simulink model "sampleModel124"  (R2021b)
settings: Solver=VariableStepAuto  StartTime=0.0  StopTime=10.0  RelTol=1e-3
undefined symbols (not defined in the file or in its folder): Newton, Raphson
libraries: simulink x7
settings Model: Creator=user  LastModifiedBy=user

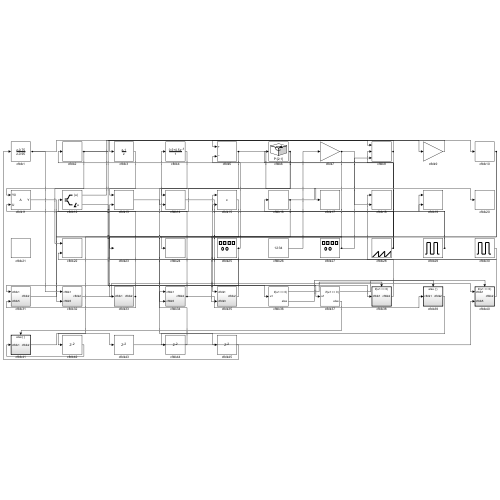
[thumbnail: Simulink's stored preview of the top-level diagram]
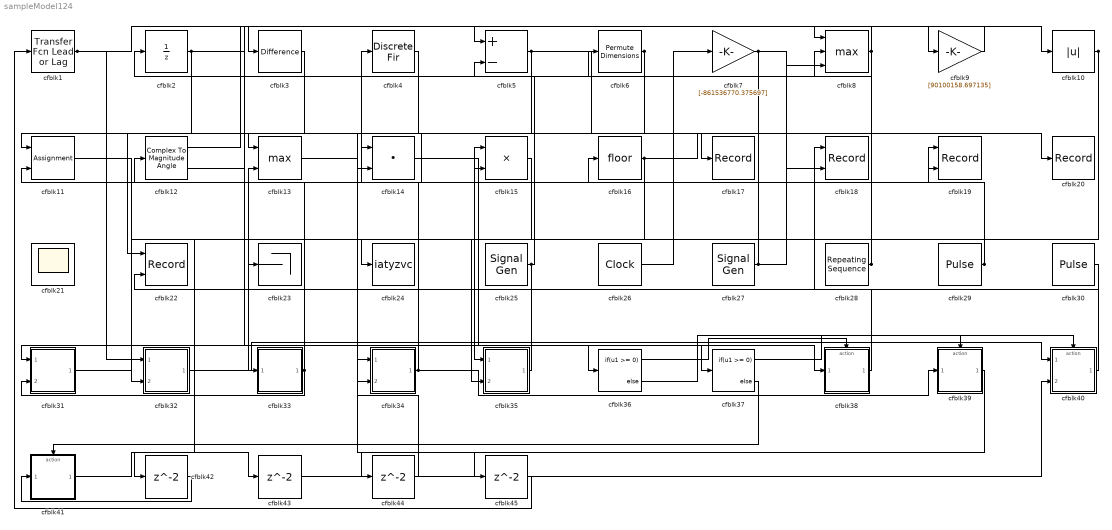
== system sampleModel124 ==
  cfblk1 : simulink/Discrete/Transfer Fcn Lead or Lag  PoleZ=0.95  ZeroZ=0.75  ICPrevOutput=0.0  ICPrevInput=0.0  DoSatur=off
      settings: SourceProductBaseCode=SL
  cfblk10 : Abs
  cfblk11 : Assignment  DiagnosticForDimensions=Warning  IndexOptions=Index vector (dialog)  Indices=1  OutputSizes=1
  cfblk12 : ComplexToMagnitudeAngle
  cfblk13 : MinMax  Function=max  Inputs=2
  cfblk14 : DotProduct  InputSameDT=on  OutDataTypeStr=Inherit: Inherit via internal rule
  cfblk15 : Product  Inputs=**
  cfblk16 : Rounding
  cfblk17 : Record  FileSettingsInternal="{\"entries\":[{\"content\":{\"excelSettings\":{\"content\":{},\"type\":\"Streamout.ExcelSettings\"}},\"type\":\"Streamout.FileSettingStorage\",\"uuid\":\"4b455be7-6192-4367-962d-3753fbca5225\"}],\"packageUris\":[\"http://schema.mathworks.com/mf0/streamout_blocks/R2020a\"],\"version\":\"1.0\"}"  SignalsInternal="{\"entries\":[{\"content\":{\"signals\":[{\"content\":{\"blockPath\":[\"sampleModel124/cfblk17\"],\"channel\":[],\"dimensions\":[1],\"domain\":\"sampleModel124/cfblk17\",\"lineColor\":\"#ff6929\",\"plots\":[1],\"port\":1,\"sid\":[\"\"],\"signalID\":4331,\"signalName\":\"cfblk5\"},\"type\":\"RecordBlkView.Signal\",\"uuid\":\"d4c4a8db-8163-4ec6-83a6-40b1eebb3f8b\"}]},\"type\":\"RecordBlkView.InputSignals\",\"uuid\":\"e1b93c3d-c5e7-46c7-8ecf-dc3223401c6b\"}],\"packageUris\":[\"http://schema.mathworks.com/mf0/streamout_blocks/R2020a\"],\"version\":\"1.0\"}"  VisualizationBindings="{\"sparklinesplugin\":{\"info\":[{\"bindingParametersList\":[],\"subplotID\":1}]}}"
  cfblk18 : Record  FileSettingsInternal="{\"entries\":[{\"content\":{\"excelSettings\":{\"content\":{},\"type\":\"Streamout.ExcelSettings\"}},\"type\":\"Streamout.FileSettingStorage\",\"uuid\":\"5ddf4468-bc94-43dd-8064-347963570ec6\"}],\"packageUris\":[\"http://schema.mathworks.com/mf0/streamout_blocks/R2020a\"],\"version\":\"1.0\"}"  Layout=[1 1]  SignalsInternal="{\"entries\":[{\"content\":{\"signals\":[{\"content\":{\"blockPath\":[\"sampleModel124/cfblk18\"],\"channel\":[],\"dimensions\":[1,1],\"domain\":\"sampleModel124/cfblk18\",\"lineColor\":\"#a2142f\",\"plots\":[1],\"port\":1,\"sid\":[\"\"],\"signalID\":4335,\"signalName\":\"cfblk38\"},\"type\":\"RecordBlkView.Signal\",\"uuid\":\"6f366cca-8914-4087-904e-589c9d18393c\"},{\"content\":{\"blockPath\":[\"sampleModel124/cfblk18\"],\"channel\":[],\"dimensions\":[1],\"domain\":\"sampleModel124/cfblk18\",\"lineColor\":\"#139fff\",\"plots\":[1],\"port\":2,\"sid\":[\"\"],\"signalID\":4339,\"signalName\":\"cfblk7\"},\"type\":\"RecordBlkView.Signal\",\"uuid\":\"3a6cb04f-8c68-44d5-8e53-ab1c3aa4fd33\"}]},\"type\":\"RecordBlkView.InputSignals\",\"uuid\":\"5846e25f-c3c2-42a3-b1e2-66c68f464335\"}],\"packageUris\":[\"http://schema.mathworks.com/mf0/streamout_blocks/R2020a\"],\"version\":\"1.0\"}"  VisualizationBindings="{\"xyplotplugin\":{\"info\":[{\"series\":[{\"bindingParametersList\":[{\"parameter\":\"X-Axis\",\"signalID\":4335,\"signalName\":\"cfblk38\"},{\"parameter\":\"Y-Axis\",\"signalID\":4339,\"signalName\":\"cfblk7\"}],\"seriesID\":22074}],\"subplotID\":1}]}}"  CompatibilityTag=XY
  cfblk19 : Record  FileSettingsInternal="{\"entries\":[{\"content\":{\"excelSettings\":{\"content\":{},\"type\":\"Streamout.ExcelSettings\"}},\"type\":\"Streamout.FileSettingStorage\",\"uuid\":\"7b857b01-50db-48e1-8f6f-10bc7bf9b4dc\"}],\"packageUris\":[\"http://schema.mathworks.com/mf0/streamout_blocks/R2020a\"],\"version\":\"1.0\"}"  Layout=[1 1]  SignalsInternal="{\"entries\":[{\"content\":{\"signals\":[{\"content\":{\"blockPath\":[\"sampleModel124/cfblk19\"],\"channel\":[],\"dimensions\":[1],\"domain\":\"sampleModel124/cfblk19\",\"lineColor\":\"#a2142f\",\"plots\":[1],\"port\":1,\"sid\":[\"\"],\"signalID\":4343,\"signalName\":\"cfblk31\"},\"type\":\"RecordBlkView.Signal\",\"uuid\":\"19b1038e-ab8c-450c-ab49-0e94919ec1bc\"},{\"content\":{\"blockPath\":[\"sampleModel124/cfblk19\"],\"channel\":[],\"dimensions\":[1],\"domain\":\"sampleModel124/cfblk19\",\"lineColor\":\"#139fff\",\"plots\":[1],\"port\":2,\"sid\":[\"\"],\"signalID\":4347,\"signalName\":\"cfblk29\"},\"type\":\"RecordBlkView.Signal\",\"uuid\":\"f751473d-f118-4cfb-b4a2-9e1d4d6e7c36\"}]},\"type\":\"RecordBlkView.InputSignals\",\"uuid\":\"40a505bf-7cac-4f73-ac44-17bad3b92167\"}],\"packageUris\":[\"http://schema.mathworks.com/mf0/streamout_blocks/R2020a\"],\"version\":\"1.0\"}"  VisualizationBindings="{\"xyplotplugin\":{\"info\":[{\"series\":[{\"bindingParametersList\":[{\"parameter\":\"X-Axis\",\"signalID\":4343,\"signalName\":\"cfblk31\"},{\"parameter\":\"Y-Axis\",\"signalID\":4347,\"signalName\":\"cfblk29\"}],\"seriesID\":56521}],\"subplotID\":1}]}}"  CompatibilityTag=XY
  cfblk2 : UnitDelay  HasFrameUpgradeWarning=on
  cfblk20 : Record  FileSettingsInternal="{\"entries\":[{\"content\":{\"excelSettings\":{\"content\":{},\"type\":\"Streamout.ExcelSettings\"}},\"type\":\"Streamout.FileSettingStorage\",\"uuid\":\"23d67973-0759-4e4c-82b0-1d8abc3ae8fa\"}],\"packageUris\":[\"http://schema.mathworks.com/mf0/streamout_blocks/R2020a\"],\"version\":\"1.0\"}"  SignalsInternal="{\"entries\":[{\"content\":{\"signals\":[{\"content\":{\"blockPath\":[\"sampleModel124/cfblk20\"],\"channel\":[],\"dimensions\":[1],\"domain\":\"sampleModel124/cfblk20\",\"lineColor\":\"#22b573\",\"plots\":[1],\"port\":1,\"sid\":[\"\"],\"signalID\":4351,\"signalName\":\"cfblk16\"},\"type\":\"RecordBlkView.Signal\",\"uuid\":\"15fb3d42-850b-41a6-83e3-28d36fd3b540\"}]},\"type\":\"RecordBlkView.InputSignals\",\"uuid\":\"34d700f9-c39a-480b-ad25-4cf78fa893c1\"}],\"packageUris\":[\"http://schema.mathworks.com/mf0/streamout_blocks/R2020a\"],\"version\":\"1.0\"}"  VisualizationBindings="{\"sparklinesplugin\":{\"info\":[{\"bindingParametersList\":[],\"subplotID\":1}]}}"
  cfblk21 : Scope
      settings: Floating=on
  cfblk22 : Record  FileSettingsInternal="{\"entries\":[{\"content\":{\"excelSettings\":{\"content\":{},\"type\":\"Streamout.ExcelSettings\"}},\"type\":\"Streamout.FileSettingStorage\",\"uuid\":\"737a1502-8c6c-4a6d-8c82-8cbccc807f05\"}],\"packageUris\":[\"http://schema.mathworks.com/mf0/streamout_blocks/R2020a\"],\"version\":\"1.0\"}"  Layout=[1 1]  SignalsInternal="{\"entries\":[{\"content\":{\"signals\":[{\"content\":{\"blockPath\":[\"sampleModel124/cfblk22\"],\"channel\":[],\"dimensions\":[1],\"domain\":\"sampleModel124/cfblk22\",\"lineColor\":\"#a2142f\",\"plots\":[1],\"port\":1,\"sid\":[\"\"],\"signalID\":4355,\"signalName\":\"cfblk2\"},\"type\":\"RecordBlkView.Signal\",\"uuid\":\"abac603e-1be2-48d2-8669-8db6971efd42\"},{\"content\":{\"blockPath\":[\"sampleModel124/cfblk22\"],\"channel\":[],\"dimensions\":[1],\"domain\":\"sampleModel124/cfblk22\",\"lineColor\":\"#139fff\",\"plots\":[1],\"port\":2,\"sid\":[\"\"],\"signalID\":4359,\"signalName\":\"cfblk30\"},\"type\":\"RecordBlkView.Signal\",\"uuid\":\"e1969516-407f-4a03-9ad4-0a79a05e62b6\"}]},\"type\":\"RecordBlkView.InputSignals\",\"uuid\":\"f08935e9-c4c2-4515-953a-f31a3825feeb\"}],\"packageUris\":[\"http://schema.mathworks.com/mf0/streamout_blocks/R2020a\"],\"version\":\"1.0\"}"  VisualizationBindings="{\"xyplotplugin\":{\"info\":[{\"series\":[{\"bindingParametersList\":[{\"parameter\":\"X-Axis\",\"signalID\":4355,\"signalName\":\"cfblk2\"},{\"parameter\":\"Y-Axis\",\"signalID\":4359,\"signalName\":\"cfblk30\"}],\"seriesID\":39126}],\"subplotID\":1}]}}"  CompatibilityTag=XY
  cfblk23 : Terminator
  cfblk24 : ToWorkspace  VariableName=iatyzvc  SaveFormat=Timeseries  SampleTime=-1
  cfblk25 : SignalGenerator  Amplitude=[-283486214.818912]  Units=rad/sec
  cfblk26 : DigitalClock
  cfblk27 : SignalGenerator  Amplitude=[346027948.126219]  Units=rad/sec
  cfblk28 : simulink/Sources/Repeating Sequence  rep_seq_t=[0 2]  rep_seq_y=[-846971032.088173, -565165640.752591]
  cfblk29 : DiscretePulseGenerator  PulseType=Time based  Amplitude=[374716888.884427]  Period=[86223942.976329]  PulseWidth=5  PhaseDelay=[2.000000]
  cfblk3 : simulink/Discrete/Difference  ICPrevInput=0.0  OutMin=[]  OutMax=[]  OutDataTypeStr=Inherit: Inherit via back propagation  OutDataType=fixdt(1, 16)  OutScaling=2^-10  DoSatur=off
  cfblk30 : DiscretePulseGenerator  PulseType=Time based  Amplitude=[921270961.664990]  Period=[2653904.390850]  PulseWidth=5  PhaseDelay=[1.000000]
  cfblk31 : Subsystem
  cfblk32 : Subsystem
  cfblk33 : Subsystem
  cfblk34 : Subsystem
  cfblk35 : Subsystem
  cfblk36 : If  IfExpression=u1 >= 0  SampleTime=1
  cfblk37 : If  IfExpression=u1 >= 0  SampleTime=1
  cfblk38 : Subsystem  TreatAsAtomicUnit=on
  cfblk39 : Subsystem  TreatAsAtomicUnit=on
  cfblk4 : DiscreteFir  SampleTime=1
  cfblk40 : Subsystem  TreatAsAtomicUnit=on
  cfblk41 : Subsystem  TreatAsAtomicUnit=on
  cfblk{42..45} (4 alike) : Delay  SampleTime=1
  cfblk5 : Sum  Inputs=+-
  cfblk6 : PermuteDimensions
  cfblk7 : Gain  Gain=[-861536770.375697]
  cfblk8 : MinMax  Function=max  Inputs=3
  cfblk9 : Gain  Gain=[90100158.697135]
  wires:
  cfblk1/1 -> cfblk32/1(cfblk1), cfblk8/1
  cfblk4/1 -> cfblk13/1
  cfblk12/1 -> cfblk10/1
  cfblk6/1 -> cfblk12/1, cfblk14/1
  cfblk32/1(cfblk2) -> cfblk40/1(cfblk1)
  cfblk25/1 -> cfblk31/1(cfblk1), cfblk5/2
  cfblk16/1 -> cfblk35/1(cfblk1), cfblk20/1
  cfblk26/1 -> cfblk7/1
  cfblk8/1 -> cfblk3/1, cfblk34/2(cfblk5)
  cfblk2/1 -> cfblk22/1, cfblk9/1, cfblk36/1
  cfblk5/1 -> cfblk17/1, cfblk14/2
  cfblk33/1(cfblk2) -> cfblk31/2(cfblk5), cfblk11/2
  cfblk14/1 -> cfblk37/1
  cfblk28/1 -> cfblk2/1, cfblk6/1, cfblk8/2, cfblk15/2
  cfblk31/1(cfblk2) -> cfblk19/1
  cfblk34/1(cfblk2) -> cfblk39/1(cfblk1), cfblk4/1
  cfblk35/1(cfblk2) -> cfblk13/2
  cfblk30/1 -> cfblk22/2
  cfblk29/1 -> cfblk19/2, cfblk16/1
  cfblk9/1 -> cfblk5/1
  cfblk7/1 -> cfblk33/1(cfblk1), cfblk18/2
  cfblk3/1 -> cfblk11/1
  cfblk27/1 -> cfblk23/1, cfblk8/3
  cfblk38/1(cfblk2) -> cfblk18/1
  cfblk11/1 -> cfblk24/1
  cfblk10/1 -> cfblk35/2(cfblk3), cfblk32/2(cfblk5)
  cfblk12/2 -> cfblk38/1(cfblk1)
  cfblk40/1(cfblk2) -> cfblk15/1
  cfblk36/1 -> cfblk38/Action
  cfblk36/2 -> cfblk39/Action
  cfblk37/1 -> cfblk40/Action
  cfblk37/2 -> cfblk41/Action
  cfblk15/1 -> cfblk42/1
  cfblk42/1 -> cfblk41/1(cfblk1)
  cfblk41/1(cfblk2) -> cfblk43/1
  cfblk43/1 -> cfblk40/2(cfblk5)
  cfblk39/1(cfblk2) -> cfblk44/1
  cfblk44/1 -> cfblk34/1(cfblk1)
  cfblk13/1 -> cfblk45/1
  cfblk45/1 -> cfblk1/1

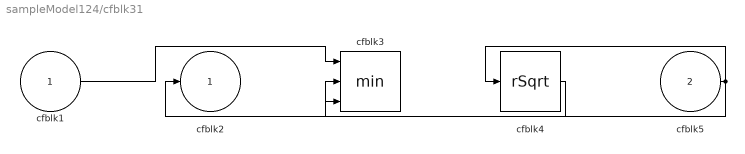
== system sampleModel124/cfblk31 ==
  cfblk1 : Inport
  cfblk5 : Inport  Port=2
  cfblk3 : MinMax  Inputs=3
  cfblk4 : Sqrt  Operator=rSqrt  AlgorithmType=Newton-Raphson  SaturateOnIntegerOverflow=on
  cfblk2 : Outport
  wires:
  cfblk5/1 -> cfblk4/1, cfblk3/2, cfblk3/3
  cfblk4/1 -> cfblk2/1
  cfblk1/1 -> cfblk3/1

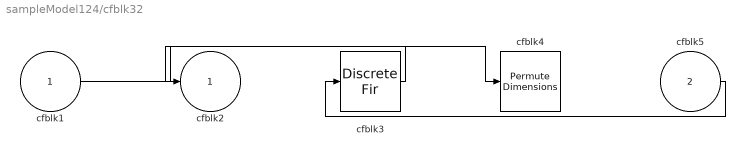
== system sampleModel124/cfblk32 ==
  cfblk1 : Inport
  cfblk5 : Inport  Port=2
  cfblk3 : DiscreteFir  SampleTime=1
  cfblk4 : PermuteDimensions
  cfblk2 : Outport
  wires:
  cfblk1/1 -> cfblk4/1
  cfblk5/1 -> cfblk3/1
  cfblk3/1 -> cfblk2/1

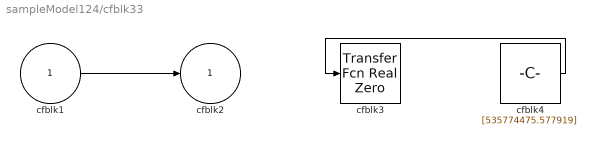
== system sampleModel124/cfblk33 ==
  cfblk1 : Inport
  cfblk3 : simulink/Discrete/Transfer Fcn Real Zero  ZeroZ=0.75  ICPrevInput=0.0  DoSatur=off
      settings: SourceProductBaseCode=SL
  cfblk4 : Constant  Value=[535774475.577919]  SampleTime=1
  cfblk2 : Outport
  wires:
  cfblk1/1 -> cfblk2/1
  cfblk4/1 -> cfblk3/1

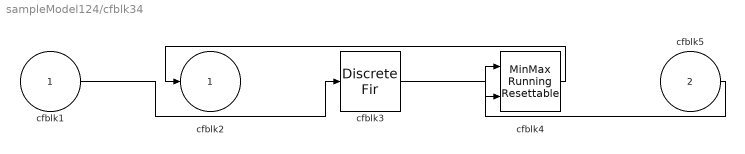
== system sampleModel124/cfblk34 ==
  cfblk1 : Inport
  cfblk5 : Inport  Port=2
  cfblk3 : DiscreteFir  SampleTime=1
  cfblk4 : simulink/Math Operations/MinMax Running Resettable  Function=min  vinit=0.0
  cfblk2 : Outport
  wires:
  cfblk4/1 -> cfblk2/1
  cfblk5/1 -> cfblk4/1
  cfblk1/1 -> cfblk3/1
  cfblk3/1 -> cfblk4/2

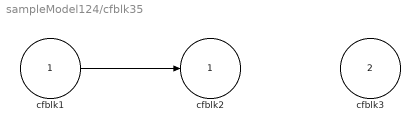
== system sampleModel124/cfblk35 ==
  cfblk1 : Inport
  cfblk3 : Inport  Port=2
  cfblk2 : Outport
  wires:
  cfblk1/1 -> cfblk2/1

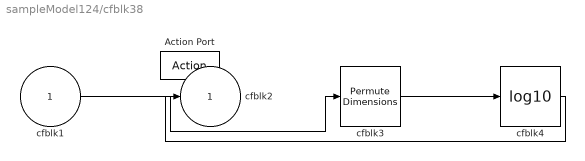
== system sampleModel124/cfblk38 ==
  cfblk1 : Inport
  Action Port : ActionPort  ActionPortLabel=if(u1 >= 0)
  cfblk3 : PermuteDimensions
  cfblk4 : Math  Operator=log10  SaturateOnIntegerOverflow=on
  cfblk2 : Outport
  wires:
  cfblk3/1 -> cfblk4/1
  cfblk1/1 -> cfblk3/1
  cfblk4/1 -> cfblk2/1

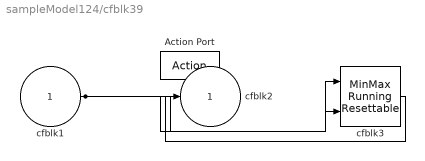
== system sampleModel124/cfblk39 ==
  cfblk1 : Inport
  Action Port : ActionPort  ActionPortLabel=else
  cfblk3 : simulink/Math Operations/MinMax Running Resettable  Function=min  vinit=0.0
  cfblk2 : Outport
  wires:
  cfblk1/1 -> cfblk3/1, cfblk3/2
  cfblk3/1 -> cfblk2/1

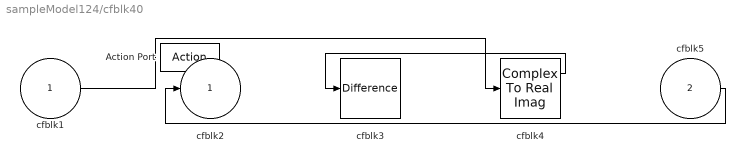
== system sampleModel124/cfblk40 ==
  cfblk1 : Inport
  cfblk5 : Inport  Port=2
  Action Port : ActionPort  ActionPortLabel=if(u1 >= 0)
  cfblk3 : simulink/Discrete/Difference  ICPrevInput=0.0  OutMin=[]  OutMax=[]  OutDataTypeStr=Inherit: Inherit via back propagation  OutDataType=fixdt(1, 16)  OutScaling=2^-10  DoSatur=off
  cfblk4 : ComplexToRealImag
  cfblk2 : Outport
  wires:
  cfblk5/1 -> cfblk2/1
  cfblk1/1 -> cfblk4/1
  cfblk4/1 -> cfblk3/1

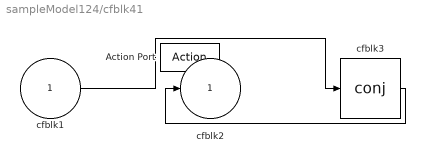
== system sampleModel124/cfblk41 ==
  cfblk1 : Inport
  Action Port : ActionPort  ActionPortLabel=else
  cfblk3 : Math  Operator=conj  SaturateOnIntegerOverflow=on
  cfblk2 : Outport
  wires:
  cfblk3/1 -> cfblk2/1
  cfblk1/1 -> cfblk3/1
